simulink model "Lab01_block"  (R2015a)
settings: Solver=ode45  StartTime=0.0  StopTime=.02  RelTol=1e-3
values from neighbouring files (symbols this model uses):
  ts = per/length(t)    [Lab01.m]
libraries: simulink x2
settings Model: Creator=robertirwin  LastModifiedBy=robertirwin

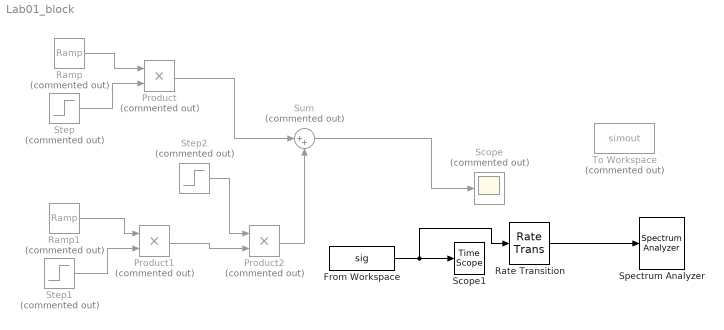
== system Lab01_block ==
  From Workspace : FromWorkspace  VariableName=sig  SampleTime=ts  Interpolate=off  OutputAfterFinalValue=Cyclic repetition
  Product : Product  Commented=on
  Product1 : Product  Commented=on
  Product2 : Product  Commented=on
  Ramp : simulink/Sources/Ramp  Commented=on  slope=10000  start=0  X0=0
  Ramp1 : simulink/Sources/Ramp  Commented=on  slope=-10000  start=.0002  X0=2
  Rate Transition : RateTransition  OutPortSampleTimeMultiple=.9
  Scope : Scope  Commented=on
  Scope1 : TimeScope
  Spectrum Analyzer : SpectrumAnalyzer
  Step : Step  Commented=on  Time=.0002  Before=1  After=0  SampleTime=0
  Step1 : Step  Commented=on  Time=.0002  SampleTime=0
  Step2 : Step  Commented=on  Time=.0006  Before=1  After=0  SampleTime=0
  Sum : Sum  Commented=on  Inputs=|++
  To Workspace : ToWorkspace  Commented=on  VariableName=simout  SaveFormat=Timeseries  SampleTime=-1
  wires:
  Step/1 -> Product/2
  Ramp/1 -> Product/1
  Product/1 -> Sum/1
  Step1/1 -> Product1/2
  Ramp1/1 -> Product1/1
  Product1/1 -> Product2/2
  Step2/1 -> Product2/1
  Product2/1 -> Sum/2
  Rate Transition/1 -> Spectrum Analyzer/1
  Sum/1 -> Scope/1
  From Workspace/1 -> Rate Transition/1, Scope1/1
